simulink model "parametric_formation_control"  (R2021a)
settings: Solver=VariableStepAuto  StartTime=0.0  StopTime=T  RelTol=1e-3
undefined symbols (not defined in the file or in its folder): params
settings Model: Creator=gaeta  LastModifiedBy=giuse
settings SolverCC: AlgebraicLoopSolver=TrustRegion
settings DataIOCC: InitialState=initialCondition  LoadInitialState=on
settings DebuggingCC: SFMachineParentedDataDiag=warning

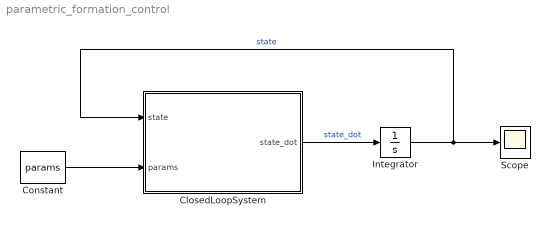
== system parametric_formation_control ==
  ClosedLoopSystem : MATLAB Function  TreatAsAtomicUnit=on
  Constant : Constant  Value=params  OutDataTypeStr=Bus: params_bus
  Integrator : Integrator
  Scope : Scope
  wires:
  Constant/1 -> ClosedLoopSystem/2(params)
  Integrator/1 -> ClosedLoopSystem/1(state), Scope/1  "state"
  ClosedLoopSystem/1(state_dot) -> Integrator/1  "state_dot"

== matlab function parametric_formation_control/ClosedLoopSystem ==
  data: state input size=6; state_dot output size=6; params input
function state_dot = closed_loop(state,params)

    n = 2;                      % task space
    N = params.N;               % number of robots
    
    p = state(1:n*N);           % robots momenta
    m = params.m;               % robots masses
    M = zeros(n*N, n*N);      	% inertia matrix
    d = params.d;               % frict. coeff
    D = zeros(n*N, n*N);        % system dissipation matrix
    for i = 1:N
        M(n*i-n+1:n*i, n*i-n+1:n*i) = eye(n).*m(i);
        D(n*i-n+1:n*i, n*i-n+1:n*i) = eye(n).*d(i);
    end
    
	E = params.E;           % number of edges
    B = params.B            % incidence matrix
    Bcl = kron(B,eye(n));	% closed-loop incidence matrix    

    z = state(n*N+1:length(state));      % edges lengths
    z_des = params.z_des;   % desired edges lengths
    dc = params.dc;         % robots dissipations
    Dc = zeros(n*E, n*E);	% controller dissipation matrix
    kc = params.kc;         % constant springs
    Kc = zeros(n*E, n*E);	% constant spring matrix
    for j = 1:E
        Dc(n*j-n+1:n*j, n*j-n+1:n*j) = eye(n).*dc(j);
        Kc(n*j-n+1:n*j, n*j-n+1:n*j) = eye(n).*kc(j);
    end

    p_dot = [-(D + Bcl*Dc*Bcl.'), -Bcl] * [M^-1*p; Kc*(z-z_des)];
    z_dot = Bcl.' * M^-1*p;

    state_dot = [p_dot; z_dot]
end




%
